simulink model "Asyncorouns"  (R2023a)
settings: Solver=VariableStepAuto  StartTime=0.0  StopTime=10.0  RelTol=1e-3
settings Model: Creator=Egypt_Laptop  LastModifiedBy=Egypt_Laptop

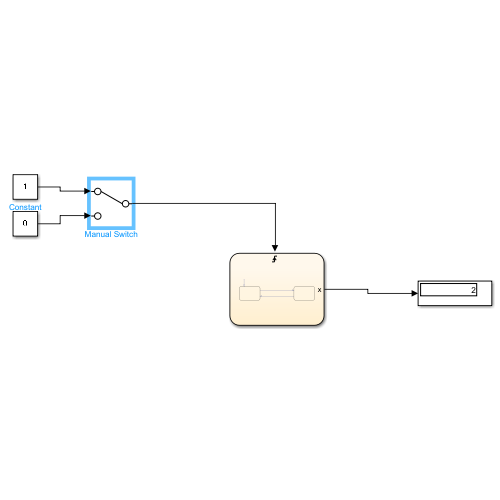
[thumbnail: Simulink's stored preview of the top-level diagram]
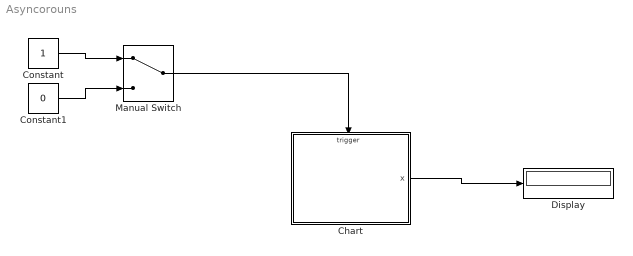
== system Asyncorouns ==
  Chart : Stateflow chart  TreatAsAtomicUnit=on
  Constant : Constant
  Constant1 : Constant  Value=0
  Display : Display
  Manual Switch : ManualSwitch
  wires:
  Manual Switch/1 -> Chart/Trigger
  Constant/1 -> Manual Switch/1
  Constant1/1 -> Manual Switch/2
  Chart/1(x) -> Display/1

== stateflow chart Asyncorouns/Chart ==
  settings: executeAtInitialization=1
  state a1
    en:
    x=1;
  state a2
    en:
    x=2;
  (default) -> a1
  a1 -> a2 : event
  a2 -> a1 : event
  data: x output
  events: event input RISING_EDGE_EVENT
